simulink model "controllore_simuilink"  (Simulink 8.3)
settings: Solver=ode45  StartTime=0.0  StopTime=300  RelTol=1e-3
values from neighbouring files (symbols this model uses):
  A = 9    [controllore.m]
  D1 = 5.5*10^(-3)    (= 0.0055)    [controllore.m]
  D2 = 5.5*10^(-3)    (= 0.0055)    [controllore.m]
  Dp = 10^(-3)    (= 0.001)    [controllore.m]
  Tp = 1    [controllore.m]
  wp = 30    [controllore.m]
libraries: cstblocks x2, simulink x2
settings Model: Creator=matdo  LastModifiedBy=matdo
settings DataIOCC: SignalLoggingSaveFormat=Dataset
settings DebuggingCC: UnderspecifiedInitializationDetection=Simplified  StateNameClashWarn=none
settings GRTTargetCC: CombineOutputUpdateFcns=on  GRTInterface=off

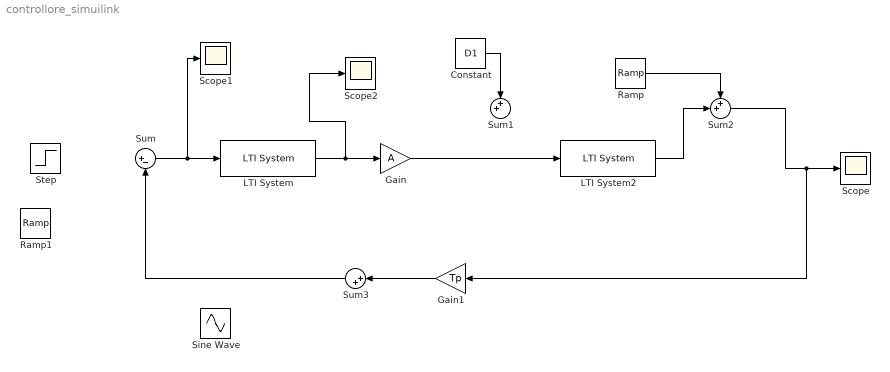
== system controllore_simuilink ==
  Constant : Constant  Value=D1
  Gain : Gain  Gain=A
  Gain1 : Gain  Gain=Tp
  LTI System : cstblocks/LTI System  sys=Ci  IC=[]
  LTI System2 : cstblocks/LTI System  sys=Gp  IC=[]
  Ramp : simulink/Sources/Ramp  slope=D2  start=0  X0=0
  Ramp1 : simulink/Sources/Ramp  slope=1  start=0  X0=0
  Scope : Scope
  Scope1 : Scope
  Scope2 : Scope
      settings: SaveName=ScopeData2
  Sine Wave : Sin  Amplitude=Dp  Frequency=wp  SampleTime=0
  Step : Step  Time=0  SampleTime=0
  Sum : Sum  Inputs=|+-
  Sum1 : Sum  Inputs=++|
  Sum2 : Sum  Inputs=++|
  Sum3 : Sum  Inputs=|++
  wires:
  Sum/1 -> Scope1/1, LTI System/1
  LTI System/1 -> Scope2/1, Gain/1
  Constant/1 -> Sum1/1
  Ramp/1 -> Sum2/1
  Gain1/1 -> Sum3/1
  Sum3/1 -> Sum/2
  Gain/1 -> LTI System2/1
  LTI System2/1 -> Sum2/2
  Sum2/1 -> Gain1/1, Scope/1
